simulink model "SVPWM21 (1)"  (R2024b)
settings: Solver=FixedStepAuto  StartTime=0.0  StopTime=0.4  RelTol=1e-3
libraries: spsIGBTDiodeLib x6, spsDCVoltageSourceLib x1, spsGroundLib x1, simulink x1, spsSeriesRLCBranchLib x1, spsThreePhaseSeriesRLCBranchLib x1, spsThreePhaseVIMeasurementLib x1, sps_lib x1
settings Model: Creator=Madhuban Computer  LastModifiedBy=Madhuban Computer
settings DataIOCC: SaveFormat=StructureWithTime  SaveOutput=off  SaveState=on  SignalLogging=off  DSMLogging=off  ReturnWorkspaceOutputs=off  LoggingToFile=on

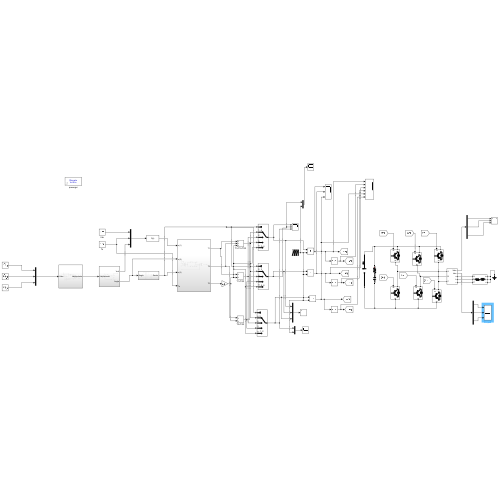
[thumbnail: Simulink's stored preview of the top-level diagram]
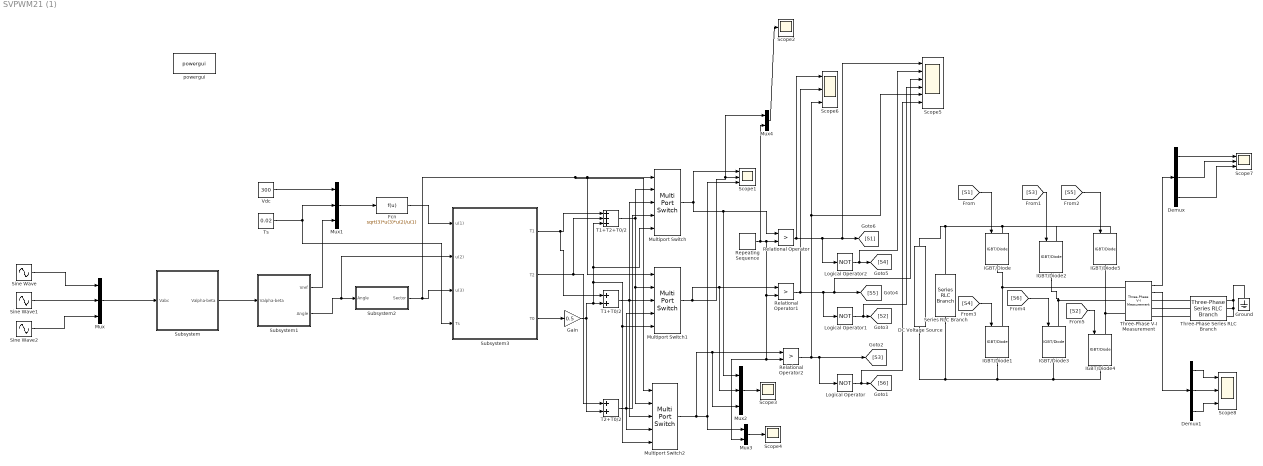
== system SVPWM21 (1) ==
  DC Voltage Source : spsDCVoltageSourceLib/DC Voltage Source  Amplitude=300  Measurements=None
  Demux : Demux  Outputs=3
  Demux1 : Demux  Outputs=3
  Fcn : Fcn  Expr=sqrt(3)*u(3)*u(2)/u(1)
  Gain : Gain  Gain=0.5
  Ground : spsGroundLib/Ground  LConnTagsString=a
  IGBT/Diode{,1..5} (6 alike) : spsIGBTDiodeLib/IGBT//Diode  Ron=1e-3  Rs=1e5  Cs=inf  Measurements=off
  Logical Operator : Logic  Operator=NOT  AllPortsSameDT=off  OutDataTypeStr=boolean
  Logical Operator1 : Logic  Operator=NOT  AllPortsSameDT=off  OutDataTypeStr=boolean
  Logical Operator2 : Logic  Operator=NOT  AllPortsSameDT=off  OutDataTypeStr=boolean
  Multiport Switch : MultiPortSwitch  DataPortOrder=Specify indices  DataPortIndices={[1,6],2,5,[3,4]}  SaturateOnIntegerOverflow=off
  Multiport Switch1 : MultiPortSwitch  DataPortOrder=Specify indices  DataPortIndices={[2,3],4,1,[5,6]}  SaturateOnIntegerOverflow=off
  Multiport Switch2 : MultiPortSwitch  DataPortOrder=Specify indices  DataPortIndices={[4,5],6,3,[1,2]}  SaturateOnIntegerOverflow=off
  Mux : Mux  Inputs=3
  Mux1 : Mux  Inputs=3
  Mux2 : Mux  Inputs=3
  Mux3 : Mux  Inputs=2
  Mux4 : Mux  Inputs=2
  Relational Operator : RelationalOperator  Operator=>  OutDataTypeStr=boolean  RndMeth=Simplest  InputSameDT=off
  Relational Operator1 : RelationalOperator  Operator=>  OutDataTypeStr=boolean  RndMeth=Simplest  InputSameDT=off
  Relational Operator2 : RelationalOperator  Operator=>  OutDataTypeStr=boolean  RndMeth=Simplest  InputSameDT=off
  Repeating Sequence : simulink/Sources/Repeating Sequence  rep_seq_t=[0 1 ]*[1/10000]  rep_seq_y=[0 0.02 ]
  Scope{1,6..8} (4 alike) : Scope  NumInputPorts=3
  Scope2 : Scope
  Scope3 : Scope
  Scope4 : Scope
  Scope5 : Scope  NumInputPorts=6
  Series RLC Branch : spsSeriesRLCBranchLib/Series RLC Branch  LConnTagsString=__new0  RConnTagsString=__new0  BranchType=RC  Resistance=0.001  Inductance=1e-3  SetiL0=off  InitialCurrent=0  Capacitance=4700e-6  Setx0=off  InitialVoltage=0  Measurements=None
  Sine Wave : Sin  Amplitude=230*0.75  Frequency=2*pi*50  SampleTime=1e-4
  Sine Wave1 : Sin  Amplitude=230*0.75  Frequency=2*pi*50  Phase=2*pi/3  SampleTime=1e-4
  Sine Wave2 : Sin  Amplitude=230*0.75  Frequency=2*pi*50  Phase=4*pi/3  SampleTime=1e-4
  Subsystem : Subsystem
  Subsystem1 : Subsystem
  Subsystem2 : Subsystem
  Subsystem3 : Subsystem
  T1+T0/2 : Sum
  T1+T2+T0/2 : Sum  Inputs=+++
  T2+T0/2 : Sum
  Three-Phase Series RLC Branch : spsThreePhaseSeriesRLCBranchLib/Three-Phase Series RLC Branch  LConnTagsString=A|B|C  RConnTagsString=A|B|C  BranchType=RL  Resistance=25  Inductance=10e-3  Capacitance=1e-6  Measurements=None
  Three-Phase V-I Measurement : spsThreePhaseVIMeasurementLib/Three-Phase V-I Measurement  VoltageMeasurement=phase-to-phase  SetLabelV=off  LabelV=Vabc  Vpu=off  VpuLL=off  CurrentMeasurement=yes  SetLabelI=off  LabelI=Iabc  Ipu=off  Pbase=100e6  Vbase=500e3  OutputType=Complex  PhasorSimulation=off  PSBequivalent=0
  Ts : Constant  Value=0.02  SampleTime=1e-4
  Vdc : Constant  Value=300
  powergui : sps_lib/powergui  Priority=1  SimulationMode=Discrete  SampleTime=1e-6  frequency=60  Iterations=50  frequencyindice=0  Pbase=100e6  ErrMax=1e-4  UnitsV=kV  UnitsW=MW  buscounter=0  FunctionMessages=off  echomessages=off  EnableUseOfTLC=off  CurrentSourceSwitches=off  DisableSnubberDevices=off  DisableRonSwitches=off  DisableVfSwitches=off  DisplayEquations=off  AutomaticDiscreteSolvers=off  SolverType=Tustin/Backward Euler (TBE)  Interpol=off  ExternalGateDelay=off  methode=off  Ts=100  x0status=blocks  SPID=on  SwTol=0  HookPort=off  NonlinearTolerance=1e-4  nMaxIteration=100  ContinueOnMaxIteration=off  RestoreLinks=warning  ResistiveCurrentMeasurement=off  Frange=[0:2:500]  Ylog=off  Xlog=on  ShowGrid=off  save=off  variable=ZData  structure=0  ZoomFFT=off  StartTime=0.0  cycles=1  DisplayStyle=1  fundamental=60  FreqAxis=off  MaxFrequency=1000  frequencyindicesteady=1  RmsSteady=1  display=off
  wires:
  Sine Wave/1 -> Mux/1
  Sine Wave1/1 -> Mux/2
  Sine Wave2/1 -> Mux/3
  Mux/1 -> Subsystem/1(Vabc)
  Subsystem/1(Valpha-beta) -> Subsystem1/1(Valpha-beta)
  Subsystem1/2(Angle) -> Subsystem3/2(u(2)), Subsystem2/1(Angle)
  Subsystem1/1(Vref) -> Mux1/3
  Vdc/1 -> Mux1/1
  Ts/1 -> Mux1/2, Subsystem3/4(Ts)
  Mux1/1 -> Fcn/1
  Fcn/1 -> Subsystem3/1(u(1))
  Subsystem2/1(Sector) -> Multiport Switch2/1, Multiport Switch1/1, Multiport Switch/1, Subsystem3/3(u(3))
  Subsystem3/3(T0) -> Gain/1
  Subsystem3/1(T1) -> T1+T2+T0/2/1, T1+T0/2/1
  Subsystem3/2(T2) -> T1+T2+T0/2/2, T2+T0/2/1
  T1+T2+T0/2/1 -> Multiport Switch/2, Multiport Switch2/2, Multiport Switch1/2
  T1+T0/2/1 -> Multiport Switch2/3, Multiport Switch1/3, Multiport Switch/3
  T2+T0/2/1 -> Multiport Switch2/4, Multiport Switch1/4, Multiport Switch/4
  Gain/1 -> Multiport Switch2/5, Multiport Switch1/5, Multiport Switch/5, T1+T2+T0/2/3, T1+T0/2/2, T2+T0/2/2
  Multiport Switch/1 -> Mux2/1, Relational Operator/1, Scope1/1
  Multiport Switch1/1 -> Mux2/2, Relational Operator1/1, Mux4/1, Scope1/2
  Multiport Switch2/1 -> Mux2/3, Relational Operator2/1, Mux3/1, Scope1/3
  Repeating Sequence/1 -> Mux4/2, Relational Operator/2, Relational Operator2/2, Mux3/2, Relational Operator1/2
  Mux2/1 -> Scope3/1
  Mux3/1 -> Scope4/1
  Relational Operator/1 -> Scope6/1, Logical Operator2/1, Scope5/1, [S1]
  Logical Operator2/1 -> Scope5/2, [S4]
  Relational Operator1/1 -> Scope6/2, Logical Operator1/1, [S5], Scope5/3
  Logical Operator1/1 -> Scope5/4, [S2]
  Relational Operator2/1 -> Scope6/3, Scope5/5, [S3], Logical Operator/1
  Logical Operator/1 -> Scope5/6, [S6]
  [S1] -> IGBT/Diode/1
  [S3] -> IGBT/Diode2/1
  [S5] -> IGBT/Diode5/1
  [S4] -> IGBT/Diode1/1
  [S6] -> IGBT/Diode3/1
  [S2] -> IGBT/Diode4/1
  Mux4/1 -> Scope2/1
  Three-Phase V-I Measurement/1 -> Demux/1
  Demux/1 -> Scope7/1
  Demux/2 -> Scope7/2
  Demux/3 -> Scope7/3
  Three-Phase V-I Measurement/2 -> Demux1/1
  Demux1/1 -> Scope8/1
  Demux1/2 -> Scope8/2
  Demux1/3 -> Scope8/3
  connections:
  IGBT/Diode/RConn1 -- Three-Phase V-I Measurement/LConn1 -- IGBT/Diode1/LConn1
  DC Voltage Source/RConn1 -- IGBT/Diode5/LConn1 -- IGBT/Diode2/LConn1 -- IGBT/Diode/LConn1 -- Series RLC Branch/LConn1
  IGBT/Diode2/RConn1 -- Three-Phase V-I Measurement/LConn2 -- IGBT/Diode3/LConn1
  IGBT/Diode4/LConn1 -- Three-Phase V-I Measurement/LConn3 -- IGBT/Diode5/RConn1
  DC Voltage Source/LConn1 -- IGBT/Diode4/RConn1 -- IGBT/Diode3/RConn1 -- IGBT/Diode1/RConn1 -- Series RLC Branch/RConn1
  Three-Phase Series RLC Branch/LConn1 -- Three-Phase V-I Measurement/RConn1
  Three-Phase Series RLC Branch/LConn2 -- Three-Phase V-I Measurement/RConn2
  Three-Phase Series RLC Branch/LConn3 -- Three-Phase V-I Measurement/RConn3
  Three-Phase Series RLC Branch/RConn1 -- Three-Phase Series RLC Branch/RConn2 -- Three-Phase Series RLC Branch/RConn3 -- Ground/LConn1

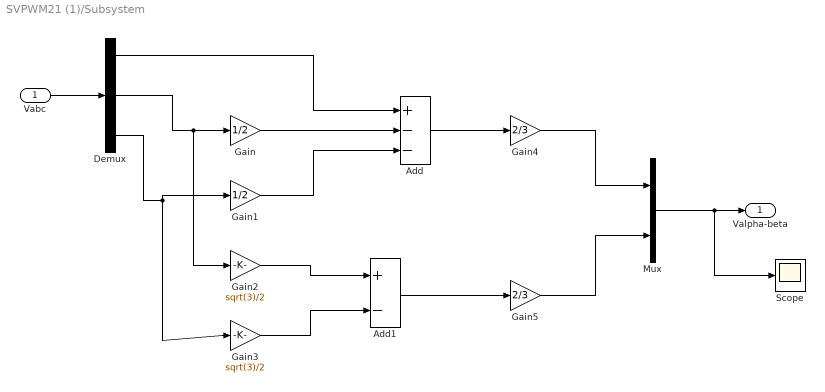
== system SVPWM21 (1)/Subsystem ==
  Vabc : Inport
  Add : Sum  Inputs=+--
  Add1 : Sum  Inputs=+-
  Demux : Demux  Outputs=3
  Gain : Gain  Gain=1/2
  Gain1 : Gain  Gain=1/2
  Gain2 : Gain  Gain=sqrt(3)/2
  Gain3 : Gain  Gain=sqrt(3)/2
  Gain4 : Gain  Gain=2/3
  Gain5 : Gain  Gain=2/3
  Mux : Mux  Inputs=2
  Scope : Scope
  Valpha-beta : Outport
  wires:
  Vabc/1 -> Demux/1
  Demux/1 -> Add/1
  Demux/2 -> Gain2/1, Gain/1
  Gain/1 -> Add/2
  Demux/3 -> Gain3/1, Gain1/1
  Gain1/1 -> Add/3
  Gain2/1 -> Add1/1
  Gain3/1 -> Add1/2
  Add/1 -> Gain4/1
  Add1/1 -> Gain5/1
  Gain5/1 -> Mux/2
  Mux/1 -> Scope/1, Valpha-beta/1
  Gain4/1 -> Mux/1

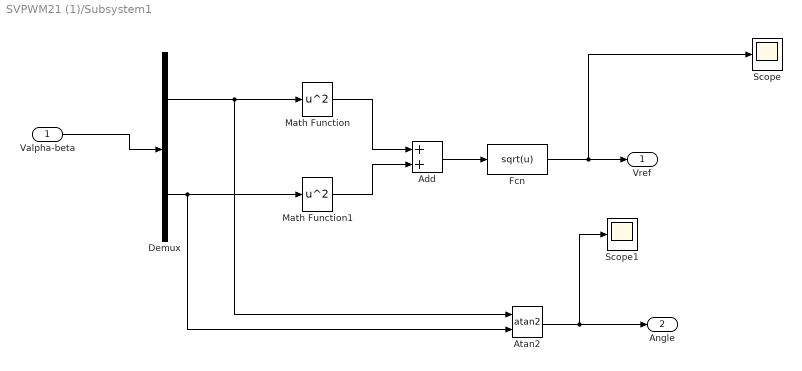
== system SVPWM21 (1)/Subsystem1 ==
  Valpha-beta : Inport
  Add : Sum
  Atan2 : Trigonometry  Operator=atan2
  Demux : Demux  Outputs=2
  Fcn : Fcn  Expr=sqrt(u)
  Math Function : Math  Operator=square  OutputSignalType=real
  Math Function1 : Math  Operator=square  OutputSignalType=real
  Scope : Scope
  Scope1 : Scope
  Vref : Outport
  Angle : Outport  Port=2
  wires:
  Valpha-beta/1 -> Demux/1
  Demux/1 -> Atan2/1, Math Function/1
  Demux/2 -> Atan2/2, Math Function1/1
  Math Function/1 -> Add/1
  Math Function1/1 -> Add/2
  Add/1 -> Fcn/1
  Fcn/1 -> Scope/1, Vref/1
  Atan2/1 -> Scope1/1, Angle/1

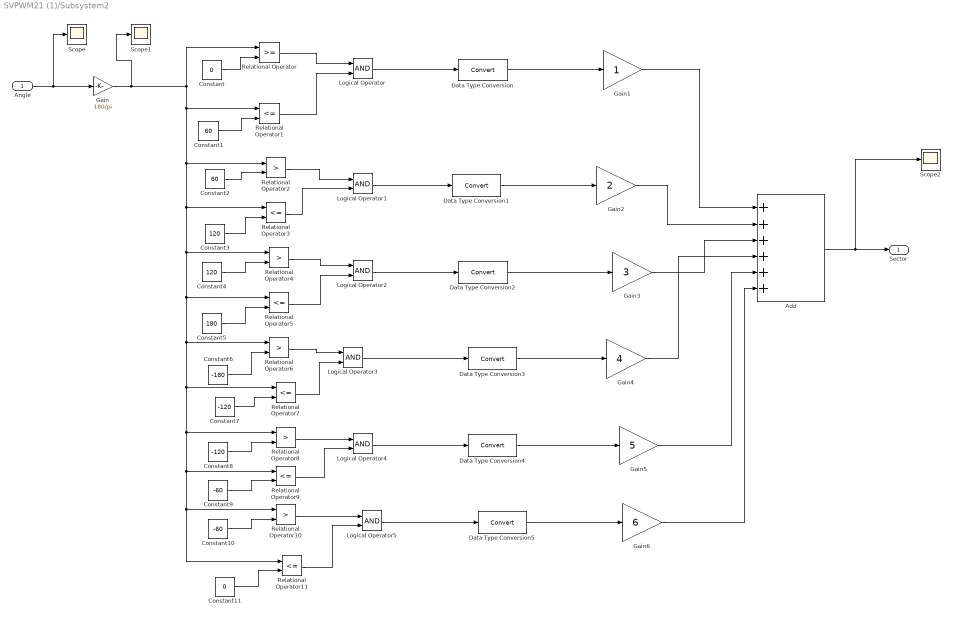
== system SVPWM21 (1)/Subsystem2 ==
  Angle : Inport
  Add : Sum  Inputs=++++++
  Constant : Constant  Value=0
  Constant1 : Constant  Value=60
  Constant10 : Constant  Value=-60
  Constant11 : Constant  Value=0
  Constant2 : Constant  Value=60
  Constant3 : Constant  Value=120
  Constant4 : Constant  Value=120
  Constant5 : Constant  Value=180
  Constant6 : Constant  Value=-180
  Constant7 : Constant  Value=-120
  Constant8 : Constant  Value=-120
  Constant9 : Constant  Value=-60
  Data Type Conversion{,1..5} (6 alike) : DataTypeConversion  SaturateOnIntegerOverflow=off  RndMeth=Floor
  Gain : Gain  Gain=180/pi
  Gain1 : Gain
  Gain2 : Gain  Gain=2
  Gain3 : Gain  Gain=3
  Gain4 : Gain  Gain=4
  Gain5 : Gain  Gain=5
  Gain6 : Gain  Gain=6
  Logical Operator{,1..5} (6 alike) : Logic  AllPortsSameDT=off  OutDataTypeStr=boolean
  Relational Operator : RelationalOperator  OutDataTypeStr=boolean  RndMeth=Simplest  InputSameDT=off
  Relational Operator{1,3,5,7,9,11} (6 alike) : RelationalOperator  Operator=<=  OutDataTypeStr=boolean  RndMeth=Simplest  InputSameDT=off
  Relational Operator{2,4,6,8,10} (5 alike) : RelationalOperator  Operator=>  OutDataTypeStr=boolean  RndMeth=Simplest  InputSameDT=off
  Scope : Scope
  Scope1 : Scope
  Scope2 : Scope
  Sector : Outport
  wires:
  Angle/1 -> Scope/1, Gain/1
  Gain/1 -> Scope1/1, Relational Operator/1, Relational Operator11/1, Relational Operator10/1, Relational Operator9/1, Relational Operator8/1, Relational Operator7/1, Relational Operator6/1, Relational Operator5/1, Relational Operator4/1, Relational Operator3/1, Relational Operator2/1, Relational Operator1/1
  Constant/1 -> Relational Operator/2
  Constant1/1 -> Relational Operator1/2
  Constant2/1 -> Relational Operator2/2
  Constant3/1 -> Relational Operator3/2
  Constant4/1 -> Relational Operator4/2
  Constant5/1 -> Relational Operator5/2
  Constant6/1 -> Relational Operator6/2
  Constant7/1 -> Relational Operator7/2
  Constant8/1 -> Relational Operator8/2
  Constant9/1 -> Relational Operator9/2
  Constant10/1 -> Relational Operator10/2
  Constant11/1 -> Relational Operator11/2
  Relational Operator/1 -> Logical Operator/1
  Relational Operator1/1 -> Logical Operator/2
  Relational Operator2/1 -> Logical Operator1/1
  Relational Operator3/1 -> Logical Operator1/2
  Relational Operator4/1 -> Logical Operator2/1
  Relational Operator5/1 -> Logical Operator2/2
  Relational Operator6/1 -> Logical Operator3/1
  Relational Operator7/1 -> Logical Operator3/2
  Relational Operator8/1 -> Logical Operator4/1
  Relational Operator9/1 -> Logical Operator4/2
  Relational Operator10/1 -> Logical Operator5/1
  Relational Operator11/1 -> Logical Operator5/2
  Logical Operator/1 -> Data Type Conversion/1
  Logical Operator1/1 -> Data Type Conversion1/1
  Logical Operator2/1 -> Data Type Conversion2/1
  Logical Operator3/1 -> Data Type Conversion3/1
  Logical Operator4/1 -> Data Type Conversion4/1
  Logical Operator5/1 -> Data Type Conversion5/1
  Data Type Conversion/1 -> Gain1/1
  Data Type Conversion1/1 -> Gain2/1
  Data Type Conversion2/1 -> Gain3/1
  Data Type Conversion3/1 -> Gain4/1
  Data Type Conversion4/1 -> Gain5/1
  Data Type Conversion5/1 -> Gain6/1
  Gain1/1 -> Add/1
  Gain2/1 -> Add/2
  Gain3/1 -> Add/3
  Gain4/1 -> Add/4
  Gain5/1 -> Add/5
  Gain6/1 -> Add/6
  Add/1 -> Scope2/1, Sector/1

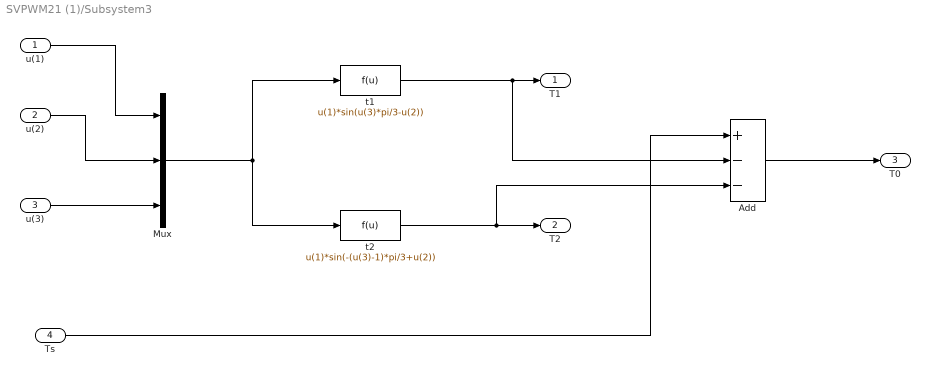
== system SVPWM21 (1)/Subsystem3 ==
  u(1) : Inport
  u(2) : Inport  Port=2
  u(3) : Inport  Port=3
  Ts : Inport  Port=4
  Add : Sum  Inputs=+--
  Mux : Mux  Inputs=3
  t1 : Fcn  Expr=u(1)*sin(u(3)*pi/3-u(2))
  t2 : Fcn  Expr=u(1)*sin(-(u(3)-1)*pi/3+u(2))
  T1 : Outport
  T2 : Outport  Port=2
  T0 : Outport  Port=3
  wires:
  u(1)/1 -> Mux/1
  u(2)/1 -> Mux/2
  u(3)/1 -> Mux/3
  Mux/1 -> t2/1, t1/1
  t1/1 -> Add/2, T1/1
  t2/1 -> Add/3, T2/1
  Ts/1 -> Add/1
  Add/1 -> T0/1
